simulink model "ac_ac_regulator"  (R2024b)
settings: Solver=VariableStepAuto  StartTime=0.0  StopTime=10.0  MaxStep=1e-4  RelTol=1e-3
undefined symbols (not defined in the file or in its folder): alpha
libraries: spsThyristorLib x2, spsVoltageMeasurementLib x2, spsACVoltageSourceLib x1, spsRMSLib x1, spsSeriesRLCBranchLib x1, sps_lib x1
settings Model: Creator=Admin  LastModifiedBy=pragy

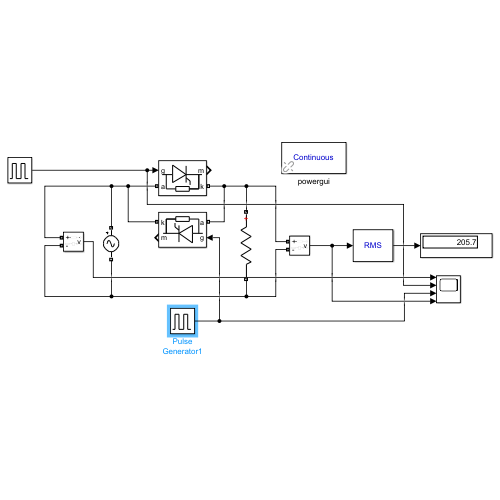
[thumbnail: Simulink's stored preview of the top-level diagram]
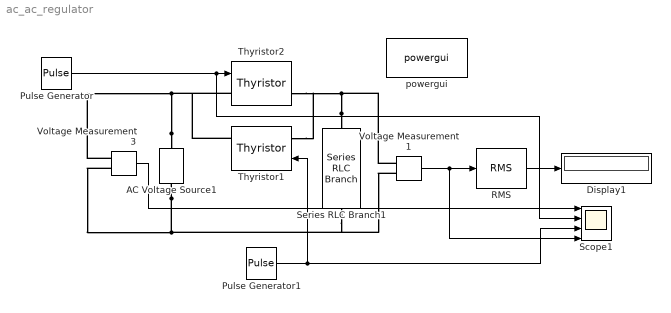
== system ac_ac_regulator ==
  AC Voltage Source1 : spsACVoltageSourceLib/AC Voltage Source  Amplitude=sqrt(2)*230  Phase=0  Frequency=50  SampleTime=0  Measurements=None  BusType=swing  Pref=10e3  Qref=0  Qmin=-inf  Qmax=+inf
  Display1 : Display
  Pulse Generator : DiscretePulseGenerator  PulseType=Time based  Period=1/50  PulseWidth=5  PhaseDelay=alpha*(0.02/360)
  Pulse Generator1 : DiscretePulseGenerator  PulseType=Time based  Period=1/50  PulseWidth=5  PhaseDelay=(180+alpha)*(0.02/360)
  RMS : spsRMSLib/RMS  TrueRMS=on  Freq=50  RMSInit=120  Ts=0
  Scope1 : Scope  NumInputPorts=4
  Series RLC Branch1 : spsSeriesRLCBranchLib/Series RLC Branch  LConnTagsString=__new0  RConnTagsString=__new0  BranchType=R  Resistance=10  Inductance=1e-3  SetiL0=off  InitialCurrent=0  Capacitance=1e-6  Setx0=off  InitialVoltage=0  Measurements=None
  Thyristor1 : spsThyristorLib/Thyristor  Ron=0.001  Lon=0  Vf=0.8  IC=0  Rs=500  Cs=250e-9  Measurements=on
  Thyristor2 : spsThyristorLib/Thyristor  Ron=0.001  Lon=0  Vf=0.8  IC=0  Rs=500  Cs=250e-9  Measurements=on
  Voltage Measurement1 : spsVoltageMeasurementLib/Voltage Measurement  PhasorSimulation=off  OutputType=Complex  PSBequivalent=0
  Voltage Measurement3 : spsVoltageMeasurementLib/Voltage Measurement  PhasorSimulation=off  OutputType=Complex  PSBequivalent=0
  powergui : sps_lib/powergui  Priority=1  SimulationMode=Continuous  SampleTime=50e-6  frequency=60  Iterations=50  frequencyindice=50  Pbase=100e6  ErrMax=1e-4  UnitsV=kV  UnitsW=MW  buscounter=0  FunctionMessages=off  echomessages=off  EnableUseOfTLC=off  CurrentSourceSwitches=off  DisableSnubberDevices=off  DisableRonSwitches=off  DisableVfSwitches=off  DisplayEquations=off  AutomaticDiscreteSolvers=off  SolverType=Tustin/Backward Euler (TBE)  Interpol=off  ExternalGateDelay=off  methode=off  Ts=100  x0status=zero  SPID=on  SwTol=0  HookPort=off  NonlinearTolerance=1e-4  nMaxIteration=100  ContinueOnMaxIteration=off  RestoreLinks=warning  ResistiveCurrentMeasurement=off  Frange=[0:2:500]  Ylog=off  Xlog=on  ShowGrid=off  save=off  variable=ZData  structure=0  ZoomFFT=off  StartTime=0.0  cycles=1  DisplayStyle=1  fundamental=60  FreqAxis=off  MaxFrequency=1000  frequencyindicesteady=1  RmsSteady=1  display=off
  wires:
  RMS/1 -> Display1/1
  Voltage Measurement3/1 -> Scope1/1
  Pulse Generator/1 -> Scope1/2, Thyristor2/1
  Voltage Measurement1/1 -> RMS/1, Scope1/4
  Pulse Generator1/1 -> Thyristor1/1, Scope1/3
  connections:
  AC Voltage Source1/LConn1 -- Series RLC Branch1/RConn1 -- Voltage Measurement1/LConn2 -- Voltage Measurement3/LConn2
  Series RLC Branch1/LConn1 -- Thyristor1/LConn1 -- Thyristor2/RConn1 -- Voltage Measurement1/LConn1
  AC Voltage Source1/RConn1 -- Thyristor1/RConn1 -- Thyristor2/LConn1 -- Voltage Measurement3/LConn1
